simulink model "torreta_anim"  (R2015a)
settings: Solver=ode3  StartTime=0.0  StopTime=100  FixedStep=delta_t  RelTol=1e-3
values from neighbouring files (symbols this model uses):
  p0 = [-8.970149e+03 8.259738e+03 0]    [interception_libre.m]
  precision = 1    [interception.m]    (also in interception_libre.m)
  sol_a = 0    [interception.m]    (also in interception_libre.m)
  sol_b = 0    [interception.m]    (also in interception_libre.m)
  sol_c = 0    [interception.m]    (also in interception_libre.m)
  T = zeros(4,4)    [interception.m]    (also in interception_libre.m)
  T_bala = [cos(acimut) -sin(acimut) 0 x0_bala; sin(acimut) cos(acimut) 0 y0_bala; 0 0 1 0; 0 0 0 1]    [interception.m]    (also in interception_libre.m)
  u_lin = (objetivo-p0)/d    [interception.m]    (also in interception_libre.m)
  v0_misil = 500    [interception.m]    (also in interception_libre.m)
undefined symbols (not defined in the file or in its folder): px_bala, py_bala
libraries: vrlib x3, simulink x2
settings Model: Creator=danir  LastModifiedBy=Iluminada

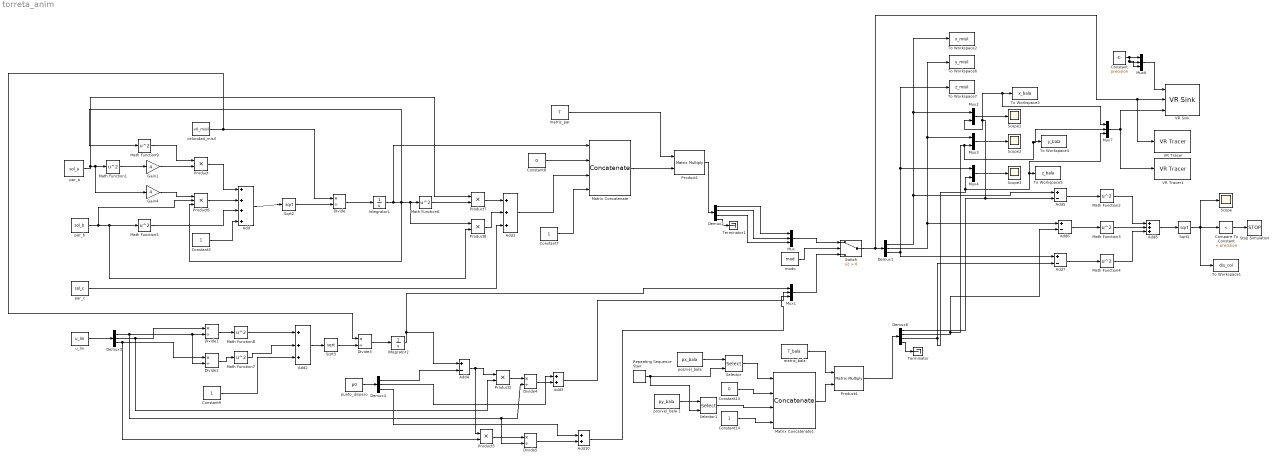
== system torreta_anim ==
  Add : Sum  Inputs=++++
  Add1 : Sum  Inputs=+++
  Add10 : Sum
  Add2 : Sum  Inputs=+++
  Add3 : Sum
  Add{4..7} (4 alike) : Sum  Inputs=+-
  Add8 : Sum  Inputs=+++
  Compare To Constant : simulink/Logic and Bit Operations/Compare To Constant  relop=<  const=precision  OutDataTypeStr=boolean
  Constant : Constant  Value=precision
  Constant13 : Constant  Tag=Elevacion  Value=0
  Constant{3,7,9,14} (4 alike) : Constant  Tag=Elevacion
  Constant8 : Constant  Tag=Elevacion  Value=0
  Demux1 : Demux  Outputs=3
  Demux2 : Demux
  Demux3 : Demux  Outputs=3
  Demux4 : Demux  Outputs=3
  Demux6 : Demux
  Divide{,1..5} (6 alike) : Product  Inputs=*/
  Gain1 : Gain  Gain=4
  Gain4 : Gain  Gain=4
  Integrator1 : Integrator
  Integrator2 : Integrator  InitialCondition=p0(1)
  Math Function{1..9} (9 alike) : Math  Operator=square  SaturateOnIntegerOverflow=on
  Matrix Concatenate : Concatenate  NumInputs=4  Mode=Multidimensional array
  Matrix Concatenate1 : Concatenate  NumInputs=4  Mode=Multidimensional array
  Mux{,1,6..7} (4 alike) : Mux  Inputs=3
  Mux2 : Mux  Inputs=2
  Mux3 : Mux  Inputs=2
  Mux4 : Mux  Inputs=2
  Product{,2..3,7..8} (5 alike) : Product
  Product1 : Product  Multiplication=Matrix(*)
  Product4 : Product  Multiplication=Matrix(*)
  Product6 : Product  Inputs=3
  Repeating Sequence Stair : simulink/Sources/Repeating Sequence Stair  OutValues=index_bala.'  tsamp=-1  OutMin=[]  OutMax=[]  OutDataTypeStr=double  OutputDataTypeScalingMode=double  OutDataType=fixdt(0,8)  ConRadixGroup=Best Precision: Vector-wise  OutScaling=2^-12
  Scope{,1..3} (4 alike) : Scope
      Scope settings: TimeRange=auto  LimitDataPoints=on  MaxDataPoints=5000  SaveToWorkspace=off  SaveName=ScopeData  YMin=93986.50188  YMax=140107.33308  SampleTime=-1  DataFormat=Array
      Scope1 settings: TimeRange=auto  LimitDataPoints=on  MaxDataPoints=5000  SaveToWorkspace=off  YMin=-10091.4526  YMax=1121.58339  SampleTime=-1  DataFormat=Array
      Scope2 settings: TimeRange=auto  LimitDataPoints=on  MaxDataPoints=5000  SaveToWorkspace=off  SaveName=ScopeData2  YMin=-1027.49282  YMax=9291.65254  SampleTime=-1  DataFormat=Array
      Scope3 settings: TimeRange=auto  LimitDataPoints=on  MaxDataPoints=5000  SaveToWorkspace=off  SaveName=ScopeData3  YMin=-624.99999  YMax=5624.99987  SampleTime=-1  DataFormat=Array
  Selector : Selector  IndexOptions=Index vector (port)  Indices=[1 3]  OutputSizes=1
  Selector1 : Selector  IndexOptions=Index vector (port)  Indices=[1 3]  OutputSizes=1
  Sqrt1 : Sqrt  SaturateOnIntegerOverflow=on
  Sqrt2 : Sqrt  SaturateOnIntegerOverflow=on
  Sqrt3 : Sqrt  SaturateOnIntegerOverflow=on
  Stop Simulation : Stop
  Switch : Switch  Criteria=u2 > Threshold
  Terminator : Terminator
  Terminator1 : Terminator
  To Workspace1 : ToWorkspace  VariableName=dis_col  SampleTime=-1
      settings: Save2DSignal=2-D array (concatenate along first dimension)
  To Workspace2 : ToWorkspace  VariableName=x_misil  SampleTime=-1
      settings: Save2DSignal=2-D array (concatenate along first dimension)
  To Workspace3 : ToWorkspace  VariableName=x_bala  SampleTime=-1
      settings: Save2DSignal=2-D array (concatenate along first dimension)
  To Workspace4 : ToWorkspace  VariableName=y_bala  SampleTime=-1
      settings: Save2DSignal=2-D array (concatenate along first dimension)
  To Workspace5 : ToWorkspace  VariableName=z_bala  SampleTime=-1
      settings: Save2DSignal=2-D array (concatenate along first dimension)
  To Workspace6 : ToWorkspace  VariableName=y_misil  SampleTime=-1
      settings: Save2DSignal=2-D array (concatenate along first dimension)
  To Workspace7 : ToWorkspace  VariableName=z_misil  SampleTime=-1
      settings: Save2DSignal=2-D array (concatenate along first dimension)
  VR Sink : vrlib/VR Sink  InstantiateOnLoad=on  SampleTime=-1  ViewEnable=on  RemoteChange=off  RemoteView=off  FieldsWritten=misil.scale.3.1.1.double#misil.translation.3.1.1.double#bala.translation.3.1.1.double  WorldFileName=robot.wrl  AutoView=off  VideoDimensions=[]  AllowVariableSize=off
  VR Tracer : vrlib/VR Tracer  VrmlFile=robot.wrl  MarkerName=Tetrahedron  UseLines=on  UseTriads=off  MarkerScale=[10 10 10]  MarkerColorSelection=Selected from color list  MarkerColor=red  rgbval=[1 0 0]  Ts=-1  ForceViewerOpen=off  ConnectPlane=off  PlaneCoeff=[0 1 0 0]  ConnectPoint=None  PointCoord=[0 0 0]
  VR Tracer1 : vrlib/VR Tracer  VrmlFile=robot.wrl  MarkerName=Pyramid  UseLines=on  UseTriads=off  MarkerScale=[10 10 10]  MarkerColorSelection=Selected from color list  MarkerColor=blue  rgbval=[1 0 0]  Ts=-1  ForceViewerOpen=off  ConnectPlane=off  PlaneCoeff=[0 1 0 0]  ConnectPoint=None  PointCoord=[0 0 0]
  matriz_bala : Constant  Tag=Elevacion  Value=T_bala  VectorParams1D=off
  "matriz_par " : Constant  Tag=Elevacion  Value=T  VectorParams1D=off
  modo : Constant  Tag=Elevacion  Value=mod
  par_a : Constant  Tag=Elevacion  Value=sol_a
  par_b : Constant  Tag=Elevacion  Value=sol_b
  par_c : Constant  Tag=Elevacion  Value=sol_c
  "pos/vel_bala " : Constant  Tag=Elevacion  Value=px_bala  VectorParams1D=off
  pos/vel_bala 1 : Constant  Tag=Elevacion  Value=py_bala  VectorParams1D=off
  punto_disparo : Constant  Tag=Elevacion  Value=p0  VectorParams1D=off
  u_lin : Constant  Tag=Elevacion  Value=u_lin
  velocidad_misil : Constant  Tag=Elevacion  Value=v0_misil
  wires:
  Add5/1 -> Math Function2/1
  Add7/1 -> Math Function4/1
  Add6/1 -> Math Function3/1
  Math Function4/1 -> Add8/3
  Math Function3/1 -> Add8/2
  Math Function2/1 -> Add8/1
  Add8/1 -> Sqrt1/1
  Sqrt1/1 -> Scope/1, To Workspace1/1, Compare To Constant/1
  Compare To Constant/1 -> Stop Simulation/1
  Mux4/1 -> Scope3/1
  Mux3/1 -> Scope2/1
  Mux2/1 -> Scope1/1
  Demux6/1 -> Add5/2, Mux7/1, To Workspace3/1, Mux2/2
  Demux6/2 -> Add6/2, Mux7/2, To Workspace4/1, Mux3/2
  Demux6/3 -> Mux4/2, Mux7/3, To Workspace5/1, Add7/2
  par_a/1 -> Product7/1, Gain4/1, Math Function1/1
  Math Function1/1 -> Gain1/1
  par_b/1 -> Product6/2, Product8/2, Math Function5/1
  Gain1/1 -> Product/2
  Gain4/1 -> Product6/1
  Product/1 -> Add/1
  Product6/1 -> Add/2
  Math Function5/1 -> Add/3
  Constant3/1 -> Add/4
  Add/1 -> Sqrt2/1
  Sqrt2/1 -> Divide/2
  Divide/1 -> Integrator1/1
  Integrator1/1 -> Matrix Concatenate/1, Product8/1, Math Function6/1, Math Function9/1, Product6/3
  Math Function6/1 -> Product7/2
  Product7/1 -> Add1/1
  Product8/1 -> Add1/2
  par_c/1 -> Add1/3
  Mux/1 -> Switch/1
  Mux1/1 -> Switch/3
  modo/1 -> Switch/2
  Switch/1 -> VR Tracer/1, VR Sink/2, Demux1/1
  Demux1/2 -> To Workspace6/1, Mux3/1, Add6/1
  Add1/1 -> Matrix Concatenate/3
  Constant7/1 -> Matrix Concatenate/4
  Constant8/1 -> Matrix Concatenate/2
  Matrix Concatenate/1 -> Product1/2
  "matriz_par "/1 -> Product1/1
  Product1/1 -> Demux2/1
  Demux2/1 -> Mux/1
  Demux2/2 -> Mux/2
  Demux2/3 -> Mux/3
  u_lin/1 -> Demux3/1
  Demux3/1 -> Divide5/2, Divide4/2, Divide2/2, Divide1/2
  Demux3/2 -> Product2/2, Divide1/1
  Demux3/3 -> Product3/2, Divide2/1
  Constant9/1 -> Add2/3
  Divide2/1 -> Math Function7/1
  Math Function7/1 -> Add2/2
  Divide1/1 -> Math Function8/1
  Math Function8/1 -> Add2/1
  Add2/1 -> Sqrt3/1
  Sqrt3/1 -> Divide3/2
  Divide3/1 -> Integrator2/1
  Integrator2/1 -> Add4/1, Mux1/1
  punto_disparo/1 -> Demux4/1
  Demux4/1 -> Add4/2
  Add4/1 -> Product3/1, Product2/1
  Product2/1 -> Divide4/1
  Divide4/1 -> Add3/2
  Demux4/2 -> Add3/1
  Product3/1 -> Divide5/1
  Divide5/1 -> Add10/2
  Demux4/3 -> Add10/1
  Add3/1 -> Mux1/2
  Add10/1 -> Mux1/3
  Constant13/1 -> Matrix Concatenate1/2
  Constant14/1 -> Matrix Concatenate1/4
  matriz_bala/1 -> Product4/1
  Matrix Concatenate1/1 -> Product4/2
  Product4/1 -> Demux6/1
  "pos/vel_bala "/1 -> Selector/1
  Demux6/4 -> Terminator/1
  Demux2/4 -> Terminator1/1
  velocidad_misil/1 -> Divide/1, Divide3/1
  Math Function9/1 -> Product/1
  Selector/1 -> Matrix Concatenate1/1
  pos/vel_bala 1/1 -> Selector1/1
  Selector1/1 -> Matrix Concatenate1/3
  Repeating Sequence Stair/1 -> Selector/2, Selector1/2
  Demux1/1 -> Add5/1, To Workspace2/1, Mux2/1
  Constant/1 -> Mux6/3, Mux6/2, Mux6/1
  Mux7/1 -> VR Tracer1/1, VR Sink/3
  Demux1/3 -> Add7/1, Mux4/1, To Workspace7/1
  Mux6/1 -> VR Sink/1
